simulink library "sm_scissor_lift_lib"  (R2017a)
settings: Solver=ode45  StartTime=0.0  StopTime=10.0  RelTol=1e-3  EnableMultiTasking=on
undefined symbols (not defined in the file or in its folder): Extr_Data_Ring, Local, X, Y, Z
undefined symbols (not defined in the file): SCL_Par
libraries: sm_lib x38, sm_scissor_lift_lib x37
(part 2 of 2)

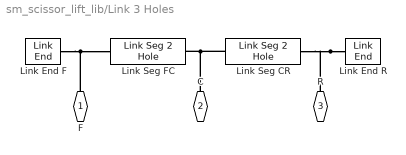
== system sm_scissor_lift_lib/Link 3 Holes ==
  Link End F : sm_scissor_lift_lib/Link End  circ_radout=W/2*1e-2  circ_radin=r*1e-2  popup_holelr=-X  deg_1=90  deg_2=270  circ_len=T*1e-2  circ_rho=rho*1e-2  circ_color=clr  circ_opc=opc
  Link End R : sm_scissor_lift_lib/Link End  circ_radout=W/2*1e-2  circ_radin=r*1e-2  popup_holelr=+X  deg_1=-90  deg_2=90  circ_len=T*1e-2  circ_rho=rho  circ_color=clr  circ_opc=opc
  Link Seg CR : sm_scissor_lift_lib/Link Seg 2 Hole  link_len=L/2*1e-2  link_width=W*1e-2  link_radh=r*1e-2  link_thickness=T*1e-2  link_rho=rho  link_color=clr  link_opc=opc
  Link Seg FC : sm_scissor_lift_lib/Link Seg 2 Hole  link_len=L/2*1e-2  link_width=W*1e-2  link_radh=r*1e-2  link_thickness=T*1e-2  link_rho=rho  link_color=clr  link_opc=opc
  F : PMIOPort  Port=1  Side=Right
  C : PMIOPort  Port=2  Side=Right
  R : PMIOPort  Port=3  Side=Right
  connections:
  Link Seg FC/RConn1 -- Link Seg CR/LConn1 -- C/RConn1
  Link End F/LConn1 -- F/RConn1 -- Link Seg FC/LConn1
  Link End R/LConn1 -- Link Seg CR/RConn1 -- R/RConn1

== system sm_scissor_lift_lib/Link End ==
  Solid : sm_lib/Body Elements/Solid  InertiaType=CalculateFromGeometry  Mass=1  MassUnits=kg  CenterOfMass=[0 0 0]  CenterOfMassUnits=m  MomentsOfInertia=[1 1 1]  MomentsOfInertiaUnits=kg*m^2  ProductsOfInertia=[0 0 0]  ProductsOfInertiaUnits=kg*m^2  DensityBased=on  Density=circ_rho  DensityUnits=kg/(m^3)  DoExposeReferenceFrame=on  SerializedFrames=<Frames/>  GraphicType=FromGeometry  MarkerShape=Sphere  MarkerSize=10  MarkerSizeUnits=m  GraphicVisPropType=SimpleVisualProperties  GraphicDiffuseColor=circ_color  GraphicSpecularColor=[0.5 0.5 0.5 1.0]  GraphicAmbientColor=[0.15 0.15 0.15 1.0]  GraphicEmissiveColor=[0.0 0.0 0.0 1.0]  GraphicShininess=75  GraphicOpacity=circ_opc  GeometryShape=GeneralExtrusion  RectangleSize=[1 1]  RectangleSizeUnits=m  BrickDimensions=[1 1 1]  BrickDimensionUnits=m  CylinderRadius=1  CylinderRadiusUnits=m  CylinderLength=1  CylinderLengthUnits=m  SphereRadius=1  SphereRadiusUnits=m  EllipsoidRadii=[1 1 1]  EllipsoidRadiiUnits=m  ExtrusionCrossSection=circ_xsec  ExtrusionCrossSectionUnits=m  ExtrusionLength=circ_len  ExtrusionLengthUnits=m  PolygonNumSides=3  PolygonOuterRadius=1  PolygonOuterRadiusUnits=m  ExtGeomFileType=STL  ExtGeomFileUnits=m  RevolutionCrossSection=[1 1; 1 -1; 2 -1; 2 1]  RevolutionCrossSectionUnits=m  RevolutionExtent=Full  RevolutionAngle=180  RevolutionAngleUnits=deg
  Transform B : sm_lib/Frames and Transforms/Rigid Transform  TranslationMethod=None  TranslationStandardOffset=0  TranslationLengthUnit=m  TranslationStandardAxis=+X  TranslationCartesianOffset=[0 0 0]  TranslationROffset=0  TranslationROffsetUnits=m  TranslationZOffset=0  TranslationZOffsetUnits=m  TranslationThetaOffset=0  TranslationThetaOffsetUnits=deg  RotationMethod=StandardAxis  RotationAngleUnits=deg  RotationStandardAxis=+Y  RotationAngle=0  RotationArbitraryAxis=[0 0 1]  FollAlignAxisA=+X  BaseAlignAxisA=+Y  FollAlignAxisB=+Y  BaseAlignAxisB=+Z  RotationSequenceAxes=FollowerAxes  RotationSequence=XYX  RotationSequenceAngles=[0 0 0]  RotationSequenceAnglesUnits=deg  RotationMatrix=[1 0 0; 0 1 0; 0 0 1]
  +X : PMIOPort  Port=1  Side=Left
  connections:
  Transform B/LConn1 -- +X/RConn1
  Transform B/RConn1 -- Solid/RConn1

== system sm_scissor_lift_lib/Link Seg 2 Hole ==
  Solid : sm_lib/Body Elements/Solid  InertiaType=CalculateFromGeometry  Mass=1  MassUnits=kg  CenterOfMass=[0 0 0]  CenterOfMassUnits=m  MomentsOfInertia=[1 1 1]  MomentsOfInertiaUnits=kg*m^2  ProductsOfInertia=[0 0 0]  ProductsOfInertiaUnits=kg*m^2  DensityBased=on  Density=link_rho  DensityUnits=kg/(m^3)  DoExposeReferenceFrame=on  SerializedFrames=<Frames/>  GraphicType=FromGeometry  MarkerShape=Sphere  MarkerSize=10  MarkerSizeUnits=m  GraphicVisPropType=SimpleVisualProperties  GraphicDiffuseColor=link_color  GraphicSpecularColor=[0.5 0.5 0.5 1.0]  GraphicAmbientColor=[0.15 0.15 0.15 1.0]  GraphicEmissiveColor=[0.0 0.0 0.0 1.0]  GraphicShininess=75  GraphicOpacity=link_opc  GeometryShape=GeneralExtrusion  RectangleSize=[1 1]  RectangleSizeUnits=m  BrickDimensions=[1 1 1]  BrickDimensionUnits=m  CylinderRadius=1  CylinderRadiusUnits=m  CylinderLength=1  CylinderLengthUnits=m  SphereRadius=1  SphereRadiusUnits=m  EllipsoidRadii=[1 1 1]  EllipsoidRadiiUnits=m  ExtrusionCrossSection=link_xsec  ExtrusionCrossSectionUnits=m  ExtrusionLength=link_thickness  ExtrusionLengthUnits=m  PolygonNumSides=3  PolygonOuterRadius=1  PolygonOuterRadiusUnits=m  ExtGeomFileType=STL  ExtGeomFileUnits=m  RevolutionCrossSection=[1 1; 1 -1; 2 -1; 2 1]  RevolutionCrossSectionUnits=m  RevolutionExtent=Full  RevolutionAngle=180  RevolutionAngleUnits=deg
  Transform B : sm_lib/Frames and Transforms/Rigid Transform  TranslationMethod=StandardAxis  TranslationStandardOffset=link_len/2  TranslationLengthUnit=m  TranslationStandardAxis=-X  TranslationCartesianOffset=[0 0 0]  TranslationROffset=0  TranslationROffsetUnits=m  TranslationZOffset=0  TranslationZOffsetUnits=m  TranslationThetaOffset=0  TranslationThetaOffsetUnits=deg  RotationMethod=None  RotationAngleUnits=deg  RotationStandardAxis=+Z  RotationAngle=0.0  RotationArbitraryAxis=[0 0 1]  FollAlignAxisA=+X  BaseAlignAxisA=+Y  FollAlignAxisB=+Y  BaseAlignAxisB=+Z  RotationSequenceAxes=FollowerAxes  RotationSequence=XYX  RotationSequenceAngles=[0 0 0]  RotationSequenceAnglesUnits=deg  RotationMatrix=[1 0 0; 0 1 0; 0 0 1]
  Transform F : sm_lib/Frames and Transforms/Rigid Transform  TranslationMethod=StandardAxis  TranslationStandardOffset=link_len/2  TranslationLengthUnit=m  TranslationStandardAxis=+X  TranslationCartesianOffset=[0 0 0]  TranslationROffset=0  TranslationROffsetUnits=m  TranslationZOffset=0  TranslationZOffsetUnits=m  TranslationThetaOffset=0  TranslationThetaOffsetUnits=deg  RotationMethod=None  RotationAngleUnits=deg  RotationStandardAxis=+Z  RotationAngle=0.0  RotationArbitraryAxis=[0 0 1]  FollAlignAxisA=+X  BaseAlignAxisA=+Y  FollAlignAxisB=+Y  BaseAlignAxisB=+Z  RotationSequenceAxes=FollowerAxes  RotationSequence=XYX  RotationSequenceAngles=[0 0 0]  RotationSequenceAnglesUnits=deg  RotationMatrix=[1 0 0; 0 1 0; 0 0 1]
  F : PMIOPort  Port=1  Side=Right
  B : PMIOPort  Port=2  Side=Left
  connections:
  Solid/RConn1 -- Transform F/LConn1 -- Transform B/LConn1
  Transform B/RConn1 -- B/RConn1
  Transform F/RConn1 -- F/RConn1

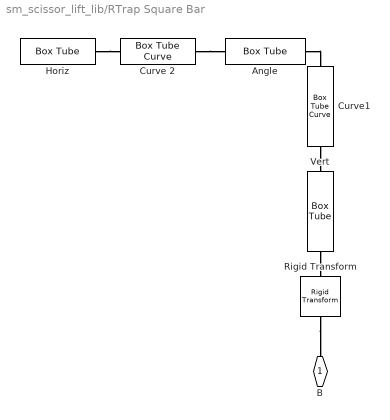
== system sm_scissor_lift_lib/RTrap Square Bar ==
  Angle : sm_scissor_lift_lib/Box Tube  box_ox=pipe_width*1e-2  box_ix=0  box_oy=pipe_width*1e-2  box_iy=0  box_len=(height_c2-height_c1)/sind(90-curve_ang1)*1e-2  box_rho=rho  box_color=clr  box_opc=1
  Curve 2 : sm_scissor_lift_lib/Box Tube Curve  box_ox=pipe_width*1e-2  box_ix=0  box_oy=pipe_width*1e-2  box_iy=0  arc_rad=rail_curve_rad1*1e-2  arc_angle=-(90-curve_ang1)  popup_arcdir=Y  box_rho=rho  box_color=clr  box_opc=1
  Curve1 : sm_scissor_lift_lib/Box Tube Curve  box_ox=pipe_width*1e-2  box_ix=0  box_oy=pipe_width*1e-2  box_iy=0  arc_rad=rail_curve_rad1*1e-2  arc_angle=-curve_ang1  popup_arcdir=Y  box_rho=rho  box_color=clr  box_opc=1
  Horiz : sm_scissor_lift_lib/Box Tube  box_ox=pipe_width*1e-2  box_ix=0  box_oy=pipe_width*1e-2  box_iy=0  box_len=((width-rail_curve_rad1-(height_c2-height_c1)/tand(90-curve_ang1)))*1e-2  box_rho=rho  box_color=clr  box_opc=1
  Rigid Transform : sm_lib/Frames and Transforms/Rigid Transform  TranslationMethod=None  TranslationStandardOffset=0  TranslationLengthUnit=m  TranslationStandardAxis=+Z  TranslationCartesianOffset=[0 0 0]  TranslationROffset=0  TranslationROffsetUnits=m  TranslationZOffset=0  TranslationZOffsetUnits=m  TranslationThetaOffset=0  TranslationThetaOffsetUnits=deg  RotationMethod=StandardAxis  RotationAngleUnits=deg  RotationStandardAxis=+Y  RotationAngle=-90  RotationArbitraryAxis=[0 0 1]  FollAlignAxisA=+X  BaseAlignAxisA=+Y  FollAlignAxisB=+Y  BaseAlignAxisB=+Z  RotationSequenceAxes=FollowerAxes  RotationSequence=XYX  RotationSequenceAngles=[0 0 0]  RotationSequenceAnglesUnits=deg  RotationMatrix=[1 0 0; 0 1 0; 0 0 1]
  Vert : sm_scissor_lift_lib/Box Tube  box_ox=pipe_width*1e-2  box_ix=0  box_oy=pipe_width*1e-2  box_iy=0  box_len=height_c1*1e-2  box_rho=rho  box_color=clr  box_opc=1
  B : PMIOPort  Port=1  Side=Right
  connections:
  Rigid Transform/LConn1 -- B/RConn1
  Vert/LConn1 -- Rigid Transform/RConn1
  Curve1/LConn1 -- Vert/RConn1
  Angle/LConn1 -- Curve1/RConn1
  Curve 2/LConn1 -- Angle/RConn1
  Horiz/LConn1 -- Curve 2/RConn1

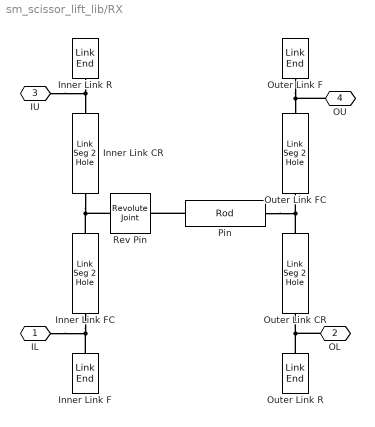
== system sm_scissor_lift_lib/RX ==
  Inner Link CR : sm_scissor_lift_lib/Link Seg 2 Hole  link_len=link_length_in/2*1e-2  link_width=link_width_in*1e-2  link_radh=link_hole_radius_in*1e-2  link_thickness=link_thickness_in*1e-2  link_rho=link_density_in  link_color=link_color_in  link_opc=link_opacity_in
  Inner Link F : sm_scissor_lift_lib/Link End  circ_radout=link_width_in/2*1e-2  circ_radin=link_hole_radius_in*1e-2  popup_holelr=-X  deg_1=90  deg_2=270  circ_len=link_thickness_in*1e-2  circ_rho=link_density_in  circ_color=link_color_in  circ_opc=link_opacity_in
  Inner Link FC : sm_scissor_lift_lib/Link Seg 2 Hole  link_len=link_length_in/2*1e-2  link_width=link_width_in*1e-2  link_radh=link_hole_radius_in*1e-2  link_thickness=link_thickness_in*1e-2  link_rho=link_density_in  link_color=link_color_in  link_opc=link_opacity_in
  Inner Link R : sm_scissor_lift_lib/Link End  circ_radout=link_width_in/2*1e-2  circ_radin=link_hole_radius_in*1e-2  popup_holelr=+X  deg_1=-90  deg_2=90  circ_len=link_thickness_in*1e-2  circ_rho=link_density_in  circ_color=link_color_in  circ_opc=link_opacity_in
  Outer Link CR : sm_scissor_lift_lib/Link Seg 2 Hole  link_len=link_length_out/2*1e-2  link_width=link_width_out*1e-2  link_radh=link_hole_radius_out*1e-2  link_thickness=link_thickness_out*1e-2  link_rho=link_density_out  link_color=link_color_out  link_opc=link_opacity_out
  Outer Link F : sm_scissor_lift_lib/Link End  circ_radout=link_width_out/2*1e-2  circ_radin=link_hole_radius_out*1e-2  popup_holelr=-X  deg_1=90  deg_2=270  circ_len=link_thickness_out*1e-2  circ_rho=link_density_out  circ_color=link_color_out  circ_opc=link_opacity_out
  Outer Link FC : sm_scissor_lift_lib/Link Seg 2 Hole  link_len=link_length_out/2*1e-2  link_width=link_width_out*1e-2  link_radh=link_hole_radius_out*1e-2  link_thickness=link_thickness_out*1e-2  link_rho=link_density_out  link_color=link_color_out  link_opc=link_opacity_out
  Outer Link R : sm_scissor_lift_lib/Link End  circ_radout=link_width_out/2*1e-2  circ_radin=link_hole_radius_out*1e-2  popup_holelr=+X  deg_1=-90  deg_2=90  circ_len=link_thickness_out*1e-2  circ_rho=link_density_out  circ_color=link_color_out  circ_opc=link_opacity_out
  Pin : sm_scissor_lift_lib/Rod  rod_rad=shaft_radius*1e-2  rod_len=shaft_length*1e-2  rod_rho=shaft_density  rod_color=shaft_color  popup_zori=Local -Z  popup_markings=None  mark_radius_range=[0.5 1.01]  mark_length_range=1.005  mark_angle_range=30  mark_color=[1 1 1]
  Rev Pin : sm_lib/Joints/Revolute Joint  SenseConstraintForce=off  SenseConstraintForceX=off  SenseConstraintForceY=off  SenseConstraintForceZ=off  SenseConstraintTorque=off  SenseConstraintTorqueX=off  SenseConstraintTorqueY=off  SenseConstraintTorqueZ=off  SenseTotalForce=off  SenseTotalForceX=off  SenseTotalForceY=off  SenseTotalForceZ=off  SenseTotalTorque=off  SenseTotalTorqueX=off  SenseTotalTorqueY=off  SenseTotalTorqueZ=off  CompositeWrenchDir=FollowerOnBase  CompositeWrenchFrame=BaseFrame  EquilibriumPosition=0  EquilibriumPositionUnits=rad  SpringStiffness=0  SpringStiffnessUnits=N*m/rad  DampingCoefficient=0  DampingCoefficientUnits=N*m/(rad/s)  TorqueActuationMode=NoTorque  MotionActuationMode=ComputedMotion  SensePosition=off  SenseVelocity=off  SenseAcceleration=off  SenseTorqueForce=off  PositionTargetSpecify=off  PositionTargetPriority=High  PositionTargetValue=0  PositionTargetValueUnits=rad  VelocityTargetSpecify=off  VelocityTargetPriority=High  VelocityTargetValue=0  VelocityTargetValueUnits=rad/s
  IL : PMIOPort  Port=1  Side=Right
  OL : PMIOPort  Port=2  Side=Right
  IU : PMIOPort  Port=3  Side=Left
  OU : PMIOPort  Port=4  Side=Left
  connections:
  Pin/RConn1 -- Rev Pin/RConn1
  Rev Pin/LConn1 -- Inner Link FC/RConn1 -- Inner Link CR/LConn1
  Inner Link F/LConn1 -- Inner Link FC/LConn1 -- IL/RConn1
  Inner Link R/LConn1 -- Inner Link CR/RConn1 -- IU/RConn1
  Outer Link CR/LConn1 -- Pin/LConn1 -- Outer Link FC/RConn1
  Outer Link R/LConn1 -- OL/RConn1 -- Outer Link CR/RConn1
  Outer Link F/LConn1 -- OU/RConn1 -- Outer Link FC/LConn1

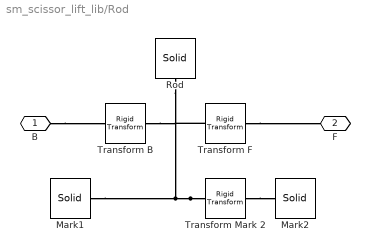
== system sm_scissor_lift_lib/Rod ==
  Mark1 : sm_lib/Body Elements/Solid  InertiaType=CalculateFromGeometry  Mass=1  MassUnits=kg  CenterOfMass=[0 0 0]  CenterOfMassUnits=m  MomentsOfInertia=[1 1 1]  MomentsOfInertiaUnits=kg*m^2  ProductsOfInertia=[1 1 1]  ProductsOfInertiaUnits=kg*m^2  DensityBased=on  Density=0  DensityUnits=kg/m^3  DoExposeReferenceFrame=on  SerializedFrames=<Frames/>  GraphicType=FromGeometry  MarkerShape=Sphere  MarkerSize=10  GraphicVisPropType=SimpleVisualProperties  GraphicDiffuseColor=mark_color  GraphicSpecularColor=[0.5 0.5 0.5 1.0]  GraphicAmbientColor=[0.15 0.15 0.15 1.0]  GraphicEmissiveColor=[0.0 0.0 0.0 1.0]  GraphicShininess=75  GraphicOpacity=mark_1_opc  GeometryShape=GeneralSolidOfRevolution  RectangleSize=[1 1]  RectangleSizeUnits=m  BrickDimensions=[1 1 1]  BrickDimensionUnits=m  CylinderRadius=1  CylinderRadiusUnits=m  CylinderLength=1  CylinderLengthUnits=m  SphereRadius=1  SphereRadiusUnits=m  EllipsoidRadii=[1 1 1]  EllipsoidRadiiUnits=m  ExtrusionCrossSection=[1 1; -1 1; -1 -1; 1 -1]  ExtrusionCrossSectionUnits=m  ExtrusionLength=1  ExtrusionLengthUnits=m  PolygonNumSides=3  PolygonOuterRadius=1  PolygonOuterRadiusUnits=m  ExtGeomFileType=STEP  ExtGeomFileUnits=m  RevolutionCrossSection=mark_xsec  RevolutionCrossSectionUnits=m  RevolutionExtent=Custom  RevolutionAngle=mark_angle_range  RevolutionAngleUnits=deg
  Mark2 : sm_lib/Body Elements/Solid  InertiaType=CalculateFromGeometry  Mass=1  MassUnits=kg  CenterOfMass=[0 0 0]  CenterOfMassUnits=m  MomentsOfInertia=[1 1 1]  MomentsOfInertiaUnits=kg*m^2  ProductsOfInertia=[1 1 1]  ProductsOfInertiaUnits=kg*m^2  DensityBased=on  Density=0  DensityUnits=kg/m^3  DoExposeReferenceFrame=on  SerializedFrames=<Frames/>  GraphicType=FromGeometry  MarkerShape=Sphere  MarkerSize=10  GraphicVisPropType=SimpleVisualProperties  GraphicDiffuseColor=mark_color  GraphicSpecularColor=[0.5 0.5 0.5 1.0]  GraphicAmbientColor=[0.15 0.15 0.15 1.0]  GraphicEmissiveColor=[0.0 0.0 0.0 1.0]  GraphicShininess=75  GraphicOpacity=mark_2_opc  GeometryShape=GeneralSolidOfRevolution  RectangleSize=[1 1]  RectangleSizeUnits=m  BrickDimensions=[1 1 1]  BrickDimensionUnits=m  CylinderRadius=1  CylinderRadiusUnits=m  CylinderLength=1  CylinderLengthUnits=m  SphereRadius=1  SphereRadiusUnits=m  EllipsoidRadii=[1 1 1]  EllipsoidRadiiUnits=m  ExtrusionCrossSection=[1 1; -1 1; -1 -1; 1 -1]  ExtrusionCrossSectionUnits=m  ExtrusionLength=1  ExtrusionLengthUnits=m  PolygonNumSides=3  PolygonOuterRadius=1  PolygonOuterRadiusUnits=m  ExtGeomFileType=STEP  ExtGeomFileUnits=m  RevolutionCrossSection=mark_xsec  RevolutionCrossSectionUnits=m  RevolutionExtent=Custom  RevolutionAngle=mark_angle_range  RevolutionAngleUnits=deg
  Rod : sm_lib/Body Elements/Solid  InertiaType=CalculateFromGeometry  Mass=1  MassUnits=kg  CenterOfMass=[0 0 0]  CenterOfMassUnits=m  MomentsOfInertia=[1 1 1]  MomentsOfInertiaUnits=kg*m^2  ProductsOfInertia=[0 0 0]  ProductsOfInertiaUnits=kg*m^2  DensityBased=on  Density=rod_rho  DensityUnits=kg/(m^3)  DoExposeReferenceFrame=on  SerializedFrames=<Frames/>  GraphicType=FromGeometry  MarkerShape=Sphere  MarkerSize=10  MarkerSizeUnits=m  GraphicVisPropType=SimpleVisualProperties  GraphicDiffuseColor=rod_color  GraphicSpecularColor=[0.5 0.5 0.5 1.0]  GraphicAmbientColor=[0.15 0.15 0.15 1.0]  GraphicEmissiveColor=[0.0 0.0 0.0 1.0]  GraphicShininess=75  GraphicOpacity=1.0  GeometryShape=Cylinder  RectangleSize=[1 1]  RectangleSizeUnits=m  BrickDimensions=[1 1 1]  BrickDimensionUnits=m  CylinderRadius=rod_rad  CylinderRadiusUnits=m  CylinderLength=rod_len  CylinderLengthUnits=m  SphereRadius=1  SphereRadiusUnits=m  EllipsoidRadii=[1 1 1]  EllipsoidRadiiUnits=m  ExtrusionCrossSection=[1 1; -1 1; -1 -1; 1 -1]  ExtrusionCrossSectionUnits=m  ExtrusionLength=1  ExtrusionLengthUnits=m  PolygonNumSides=3  PolygonOuterRadius=1  PolygonOuterRadiusUnits=m  ExtGeomFileType=STL  ExtGeomFileUnits=m  RevolutionCrossSection=[1 1; 1 -1; 2 -1; 2 1]  RevolutionCrossSectionUnits=m  RevolutionExtent=Full  RevolutionAngle=180  RevolutionAngleUnits=deg
  Transform Mark 2 : sm_lib/Frames and Transforms/Rigid Transform  TranslationMethod=None  TranslationStandardOffset=0  TranslationLengthUnit=m  TranslationStandardAxis=+Z  TranslationCartesianOffset=[0 0 0]  TranslationROffset=0  TranslationROffsetUnits=m  TranslationZOffset=0  TranslationZOffsetUnits=m  TranslationThetaOffset=0  TranslationThetaOffsetUnits=deg  RotationMethod=StandardAxis  RotationAngleUnits=deg  RotationStandardAxis=+Z  RotationAngle=180  RotationArbitraryAxis=[0 0 1]  FollAlignAxisA=+X  BaseAlignAxisA=+Y  FollAlignAxisB=+Y  BaseAlignAxisB=+Z  RotationSequenceAxes=FollowerAxes  RotationSequence=XYX  RotationSequenceAngles=[0 0 0]  RotationSequenceAnglesUnits=deg  RotationMatrix=[1 0 0; 0 1 0; 0 0 1]
  Transform B : sm_lib/Frames and Transforms/Rigid Transform  TranslationMethod=StandardAxis  TranslationStandardOffset=rod_len/2*z_ori  TranslationLengthUnit=m  TranslationStandardAxis=+Z  TranslationCartesianOffset=[0 0 0]  TranslationROffset=0  TranslationROffsetUnits=m  TranslationZOffset=0  TranslationZOffsetUnits=m  TranslationThetaOffset=0  TranslationThetaOffsetUnits=deg  RotationMethod=None  RotationAngleUnits=deg  RotationStandardAxis=+Z  RotationAngle=0.0  RotationArbitraryAxis=[0 0 1]  FollAlignAxisA=+X  BaseAlignAxisA=+Y  FollAlignAxisB=+Y  BaseAlignAxisB=+Z  RotationSequenceAxes=FollowerAxes  RotationSequence=XYX  RotationSequenceAngles=[0 0 0]  RotationSequenceAnglesUnits=deg  RotationMatrix=[1 0 0; 0 1 0; 0 0 1]
  Transform F : sm_lib/Frames and Transforms/Rigid Transform  TranslationMethod=StandardAxis  TranslationStandardOffset=rod_len/2*z_ori  TranslationLengthUnit=m  TranslationStandardAxis=+Z  TranslationCartesianOffset=[0 0 0]  TranslationROffset=0  TranslationROffsetUnits=m  TranslationZOffset=0  TranslationZOffsetUnits=m  TranslationThetaOffset=0  TranslationThetaOffsetUnits=deg  RotationMethod=None  RotationAngleUnits=deg  RotationStandardAxis=+Z  RotationAngle=0.0  RotationArbitraryAxis=[0 0 1]  FollAlignAxisA=+X  BaseAlignAxisA=+Y  FollAlignAxisB=+Y  BaseAlignAxisB=+Z  RotationSequenceAxes=FollowerAxes  RotationSequence=XYX  RotationSequenceAngles=[0 0 0]  RotationSequenceAnglesUnits=deg  RotationMatrix=[1 0 0; 0 1 0; 0 0 1]
  B : PMIOPort  Port=1  Side=Left
  F : PMIOPort  Port=2  Side=Right
  connections:
  Transform F/RConn1 -- F/RConn1
  B/RConn1 -- Transform B/LConn1
  Transform Mark 2/RConn1 -- Mark2/RConn1
  Transform Mark 2/LConn1 -- Mark1/RConn1 -- Transform F/LConn1 -- Transform B/RConn1 -- Rod/RConn1

== system sm_scissor_lift_lib/Shaft ==
  Shaft : sm_lib/Body Elements/Solid  InertiaType=CalculateFromGeometry  Mass=1  MassUnits=kg  CenterOfMass=[0 0 0]  CenterOfMassUnits=m  MomentsOfInertia=[1 1 1]  MomentsOfInertiaUnits=kg*m^2  ProductsOfInertia=[0 0 0]  ProductsOfInertiaUnits=kg*m^2  DensityBased=on  Density=Ro  DensityUnits=kg/m^3  DoExposeReferenceFrame=on  SerializedFrames=<Frames/>  GraphicType=FromGeometry  MarkerShape=Sphere  MarkerSize=1  MarkerSizeUnits=m  GraphicVisPropType=SimpleVisualProperties  GraphicDiffuseColor=clr  GraphicSpecularColor=[0.2 0.2 0.2]  GraphicAmbientColor=[0.5 0.5 0.5]  GraphicEmissiveColor=[0.1 0.1 0.1]  GraphicShininess=24.0  GraphicOpacity=opc  GeometryShape=Cylinder  RectangleSize=[1 1]  RectangleSizeUnits=m  BrickDimensions=[1 1 1]  BrickDimensionUnits=m  CylinderRadius=r  CylinderRadiusUnits=cm  CylinderLength=L  CylinderLengthUnits=cm  SphereRadius=1  SphereRadiusUnits=m  EllipsoidRadii=[1 1 1]  EllipsoidRadiiUnits=m  ExtrusionCrossSection=[1 1; -1 1; -1 -1; 1 -1]  ExtrusionCrossSectionUnits=m  ExtrusionLength=1  ExtrusionLengthUnits=m  PolygonNumSides=1  PolygonOuterRadius=1  PolygonOuterRadiusUnits=m  ExtGeomFileType=STEP  ExtGeomFileUnits=m  RevolutionCrossSection=[1 1; 1 -1; 2 -1; 2 1]  RevolutionCrossSectionUnits=m  RevolutionExtent=Full  RevolutionAngle=180  RevolutionAngleUnits=deg
  Transform ShaftCtr : sm_lib/Frames and Transforms/Rigid Transform  TranslationMethod=Cartesian  TranslationStandardOffset=0  TranslationLengthUnit=cm  TranslationStandardAxis=+Z  TranslationCartesianOffset=[0 0 L/2]*z_ori  TranslationROffset=0  TranslationROffsetUnits=m  TranslationZOffset=0  TranslationZOffsetUnits=m  TranslationThetaOffset=0  TranslationThetaOffsetUnits=deg  RotationMethod=StandardAxis  RotationAngleUnits=deg  RotationStandardAxis=+Z  RotationAngle=theta  RotationArbitraryAxis=[0 0 1]  FollAlignAxisA=+X  BaseAlignAxisA=+Y  FollAlignAxisB=+Y  BaseAlignAxisB=+Z  RotationSequenceAxes=FollowerAxes  RotationSequence=XYX  RotationSequenceAngles=[0 0 0]  RotationSequenceAnglesUnits=deg  RotationMatrix=[1 0 0; 0 1 0; 0 0 1]
  Transform ShaftF : sm_lib/Frames and Transforms/Rigid Transform  TranslationMethod=Cartesian  TranslationStandardOffset=0  TranslationLengthUnit=cm  TranslationStandardAxis=+Z  TranslationCartesianOffset=[0 0 L/2]*z_ori  TranslationROffset=0  TranslationROffsetUnits=m  TranslationZOffset=0  TranslationZOffsetUnits=m  TranslationThetaOffset=0  TranslationThetaOffsetUnits=deg  RotationMethod=None  RotationAngleUnits=deg  RotationStandardAxis=+Z  RotationAngle=0  RotationArbitraryAxis=[0 0 1]  FollAlignAxisA=+X  BaseAlignAxisA=+Y  FollAlignAxisB=+Y  BaseAlignAxisB=+Z  RotationSequenceAxes=FollowerAxes  RotationSequence=XYX  RotationSequenceAngles=[0 0 0]  RotationSequenceAnglesUnits=deg  RotationMatrix=[1 0 0; 0 1 0; 0 0 1]
  B : PMIOPort  Port=1  Side=Left
  F : PMIOPort  Port=2  Side=Right
  connections:
  Transform ShaftCtr/LConn1 -- B/RConn1
  F/RConn1 -- Transform ShaftF/RConn1
  Shaft/RConn1 -- Transform ShaftF/LConn1 -- Transform ShaftCtr/RConn1

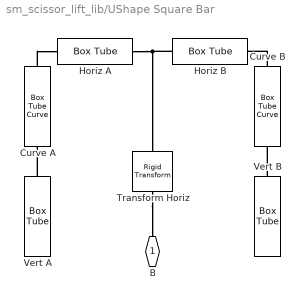
== system sm_scissor_lift_lib/UShape Square Bar ==
  Curve A : sm_scissor_lift_lib/Box Tube Curve  box_ox=pipe_width*1e-2  box_ix=0  box_oy=pipe_width*1e-2  box_iy=0  arc_rad=rail_curve_rad*1e-2  arc_angle=90  popup_arcdir=Y  box_rho=rho  box_color=clr  box_opc=1
  Curve B : sm_scissor_lift_lib/Box Tube Curve  box_ox=pipe_width*1e-2  box_ix=0  box_oy=pipe_width*1e-2  box_iy=0  arc_rad=rail_curve_rad*1e-2  arc_angle=90  popup_arcdir=Y  box_rho=rho  box_color=clr  box_opc=1
  Horiz A : sm_scissor_lift_lib/Box Tube  box_ox=pipe_width*1e-2  box_ix=0  box_oy=pipe_width*1e-2  box_iy=0  box_len=(width-rail_curve_rad*2-pipe_width*3)/2*1e-2  box_rho=rho  box_color=clr  box_opc=1
  Horiz B : sm_scissor_lift_lib/Box Tube  box_ox=pipe_width*1e-2  box_ix=0  box_oy=pipe_width*1e-2  box_iy=0  box_len=(width-rail_curve_rad*2-pipe_width*3)/2*1e-2  box_rho=rho  box_color=clr  box_opc=1
  Transform Horiz : sm_lib/Frames and Transforms/Rigid Transform  TranslationMethod=StandardAxis  TranslationStandardOffset=height  TranslationLengthUnit=cm  TranslationStandardAxis=+Z  TranslationCartesianOffset=[0 0 0]  TranslationROffset=0  TranslationROffsetUnits=m  TranslationZOffset=0  TranslationZOffsetUnits=m  TranslationThetaOffset=0  TranslationThetaOffsetUnits=deg  RotationMethod=None  RotationAngleUnits=deg  RotationStandardAxis=+Y  RotationAngle=90.0  RotationArbitraryAxis=[0 0 1]  FollAlignAxisA=+X  BaseAlignAxisA=+Y  FollAlignAxisB=+Y  BaseAlignAxisB=+Z  RotationSequenceAxes=FollowerAxes  RotationSequence=XYX  RotationSequenceAngles=[0 0 0]  RotationSequenceAnglesUnits=deg  RotationMatrix=[1 0 0; 0 1 0; 0 0 1]
  Vert A : sm_scissor_lift_lib/Box Tube  box_ox=pipe_width*1e-2  box_ix=0  box_oy=pipe_width*1e-2  box_iy=0  box_len=(height-rail_curve_rad)*1e-2  box_rho=rho  box_color=clr  box_opc=1
  Vert B : sm_scissor_lift_lib/Box Tube  box_ox=pipe_width*1e-2  box_ix=0  box_oy=pipe_width*1e-2  box_iy=0  box_len=(height-rail_curve_rad)*1e-2  box_rho=rho  box_color=clr  box_opc=1
  B : PMIOPort  Port=1  Side=Right
  connections:
  Transform Horiz/LConn1 -- B/RConn1
  Horiz B/LConn1 -- Horiz A/RConn1 -- Transform Horiz/RConn1
  Curve B/LConn1 -- Horiz B/RConn1
  Vert B/LConn1 -- Curve B/RConn1
  Curve A/RConn1 -- Horiz A/LConn1
  Vert A/RConn1 -- Curve A/LConn1
